simulink model "samples10ANC"  (R2023b)
settings: Solver=FixedStepAuto  StartTime=0.0  StopTime=inf  RelTol=1e-3
model workspace (MAT data in the model file):
  SpF = 10
libraries: matrix_library x22, dspadpt3 x20, raspberrypiAVlib x2, dspfdesign x2
settings Model: ExtModeTrigDuration=2  Creator=aaron  LastModifiedBy=aaron
settings SolverCC: PositivePriorityOrder=on  AutoInsertRateTranBlk=on
settings OptimizationCC: EnhancedBackFolding=on  PassReuseOutputArgsAs=Individual arguments  ZeroExternalMemoryAtStartup=off  ZeroInternalMemoryAtStartup=off  MaxStackSize=64  OptimizeBlockOrder=speed  DifferentSizesBufferReuse=on  OptimizationCustomize=off  EfficientTunableParamExpr=on
settings DebuggingCC: ParameterTunabilityLossMsg=error
settings HardwareCC: ProdBitPerPointer=32  ProdBitPerSizeT=32  ProdBitPerPtrDiffT=32  ProdLargestAtomicInteger=Long  ProdLargestAtomicFloat=Double  ProdWordSize=32  ProdLongLongMode=on  ProdHWDeviceType=ARM Compatible->ARM Cortex
settings RTWCC: Description=Embedded Coder  SystemTargetFile=ert.tlc  HardwareBoard=Raspberry Pi  TLCOptions="-aInlineSetEventsForThisBaseRateFcn=TLC_FALSE -aSuppressMultiTaskScheduler=TLC_FALSE  -aRateBasedStepFcn=0"  TemplateMakefile=ert_default_tmf  Toolchain=GNU GCC Embedded Linux  BuildConfiguration=Faster Runs
settings CodeAppCC: ForceParamTrailComments=on  IgnoreCustomStorageClasses=off  OperatorAnnotations=on  SimulinkDataObjDesc=on  SFDataObjDesc=on  InsertBlockDesc=on
settings ERTTargetCC: SupportVariableSizeSignals=on  ExtModeTransport=2  ExtModeStaticAlloc=on  ExtModeMexFile=ext_xcp  ExtModeIntrfLevel=Level2 - Open

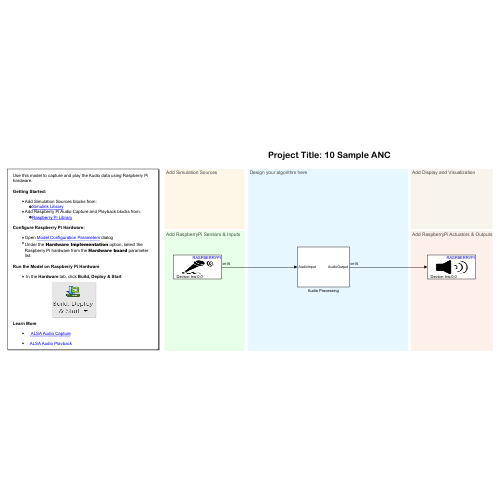
[thumbnail: Simulink's stored preview of the top-level diagram]
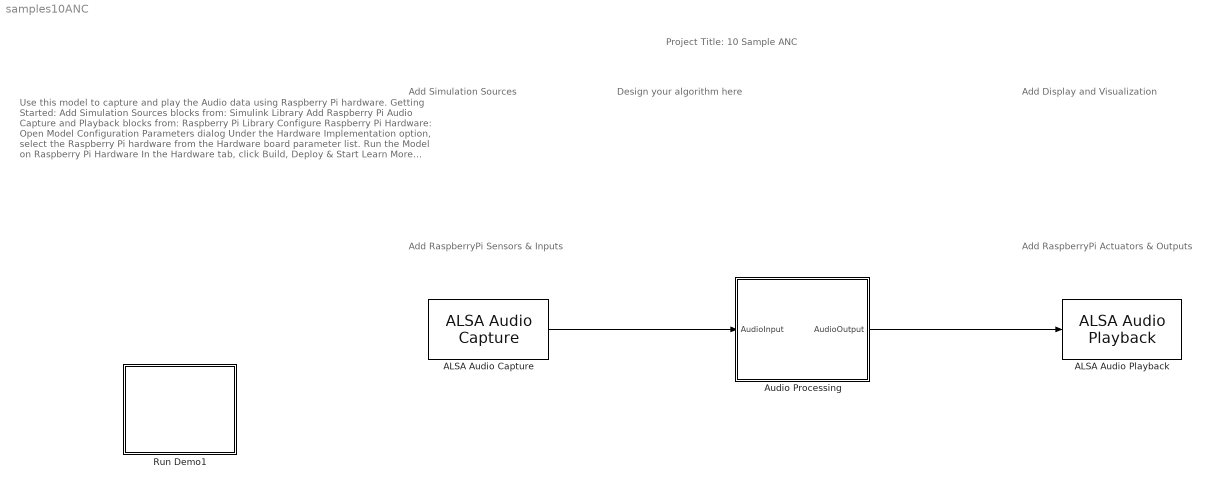
== system samples10ANC ==
  note: Project Title: 10 Sample ANC
  note: Add RaspberryPi Sensors & Inputs
  note: Add Display and Visualization
  note: Add Simulation Sources
  note: Use this model to capture and play the Audio data using Raspberry Pi hardware.
      |
      | Getting Started:
      |
      | Add Simulation Sources blocks from:
      | Simulink Library
      | Add Raspberry Pi Audio Capture and Playback blocks from:
      | Raspberry Pi Library
      |
      | Configure Raspberry Pi Hardware:
      |
      | Open Model Configuration Parameters dialog
      | Under the Hardware Implementation option, select the Raspberry Pi hardware from the Hardware board parameter list.
      |
      | Run the Model on Raspberry Pi Hardware
      |
      | In the Hardware tab, click Build, Deploy & Start
      |
      | Learn More
      | ALSA Audio Capture
      | ALSA Audio Playback
  note: Add RaspberryPi Actuators & Outputs
  note: Design your algorithm here
  ALSA Audio Capture : raspberrypiAVlib/ALSA Audio Capture  deviceStr='hw:0,0'  DataBitDepth=16-bit integer  numberOfChannels=2  sampleRateEnum=44100  frameSize=SpF  QueueDuration=0.5  blockPlatform=Raspberry Pi
  ALSA Audio Playback : raspberrypiAVlib/ALSA Audio Playback  deviceStr='hw:0,0'  sampleRateEnum=44100  queueDuration=0.5  blockPlatform=Raspberry Pi
  Audio Processing : Subsystem
  Run Demo1 : Subsystem  Description=Controls host-side RTDX processing.
      mask Display: pic=imread('raspberrypiBuildDeployAndStart.png');image(pic);
  wires:
  Audio Processing/1(AudioOutput) -> ALSA Audio Playback/1
  ALSA Audio Capture/1 -> Audio Processing/1(AudioInput)

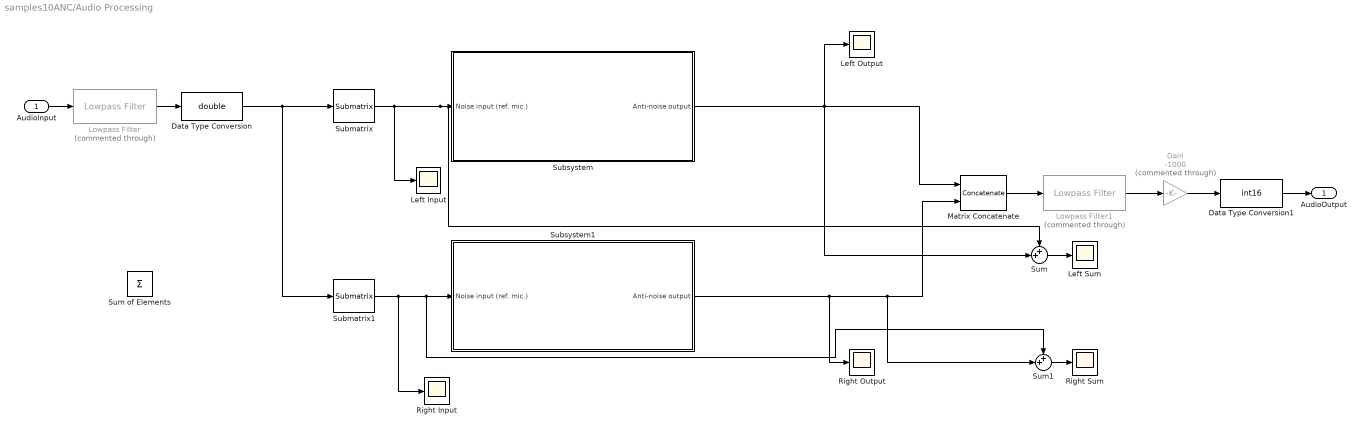
== system samples10ANC/Audio Processing ==
  AudioInput : Inport
  Data Type Conversion : DataTypeConversion  OutDataTypeStr=double  SaturateOnIntegerOverflow=off  RndMeth=Floor
  Data Type Conversion1 : DataTypeConversion  OutDataTypeStr=int16  SaturateOnIntegerOverflow=off  RndMeth=Floor  LockScale=on
  Gain : Gain  Commented=through  Gain=-1000
  Left Input : Scope
  Left Output : Scope
  Left Sum : Scope
  Lowpass Filter : dspfdesign/Lowpass Filter  Commented=through  FilterType=FIR  DesignForMinimumOrder=on  FilterOrder=50  PassbandFrequency=6e2  StopbandFrequency=10e2  PassbandRipple=0.1  StopbandAttenuation=80  SampleRateMode=Specify on dialog  SampleRate=44100  SimulateUsing=Interpreted execution  roundingMode=Floor  coeffsDataTypeStr=fixdt(1,16)
  Lowpass Filter1 : dspfdesign/Lowpass Filter  Commented=through  FilterType=FIR  DesignForMinimumOrder=on  FilterOrder=50  PassbandFrequency=6e2  StopbandFrequency=10e2  PassbandRipple=0.1  StopbandAttenuation=80  SampleRateMode=Specify on dialog  SampleRate=44100  SimulateUsing=Interpreted execution  roundingMode=Floor  coeffsDataTypeStr=fixdt(1,16)
  Matrix Concatenate : Concatenate  Mode=Multidimensional array  ConcatenateDimension=2
  Right Input : Scope
  Right Output : Scope
  Right Sum : Scope
  Submatrix : matrix_library/Submatrix  RowSpan=All rows  RowStartMode=First  RowStartIndex=1  RowEndMode=Last  RowEndIndex=1  ColSpan=One column  ColStartMode=First  ColStartIndex=1  ColEndMode=Last  ColEndIndex=1
  Submatrix1 : matrix_library/Submatrix  RowSpan=All rows  RowStartMode=First  RowStartIndex=1  RowEndMode=Last  RowEndIndex=1  ColSpan=One column  ColStartMode=Last  ColStartIndex=1  ColEndMode=Last  ColEndIndex=1
  Subsystem : Subsystem  TreatAsAtomicUnit=on
  Subsystem1 : Subsystem  TreatAsAtomicUnit=on
  Sum : Sum  Inputs=++|
  Sum of Elements : Sum  Inputs=+
  Sum1 : Sum  Inputs=++|
  AudioOutput : Outport
  wires:
  Data Type Conversion/1 -> Submatrix1/1, Submatrix/1
  Submatrix/1 -> Sum/1, Subsystem/1(Noise input (ref. mic.)), Left Input/1
  AudioInput/1 -> Lowpass Filter/1
  Submatrix1/1 -> Sum1/1, Subsystem1/1(Noise input (ref. mic.)), Right Input/1
  Subsystem1/1(Anti-noise output) -> Sum1/2, Matrix Concatenate/2, Right Output/1
  Lowpass Filter/1 -> Data Type Conversion/1
  Gain/1 -> Data Type Conversion1/1
  Lowpass Filter1/1 -> Gain/1
  Data Type Conversion1/1 -> AudioOutput/1
  Matrix Concatenate/1 -> Lowpass Filter1/1
  Sum1/1 -> Right Sum/1
  Subsystem/1(Anti-noise output) -> Sum/2, Left Output/1, Matrix Concatenate/1
  Sum/1 -> Left Sum/1

== system samples10ANC/Run Demo1 ==

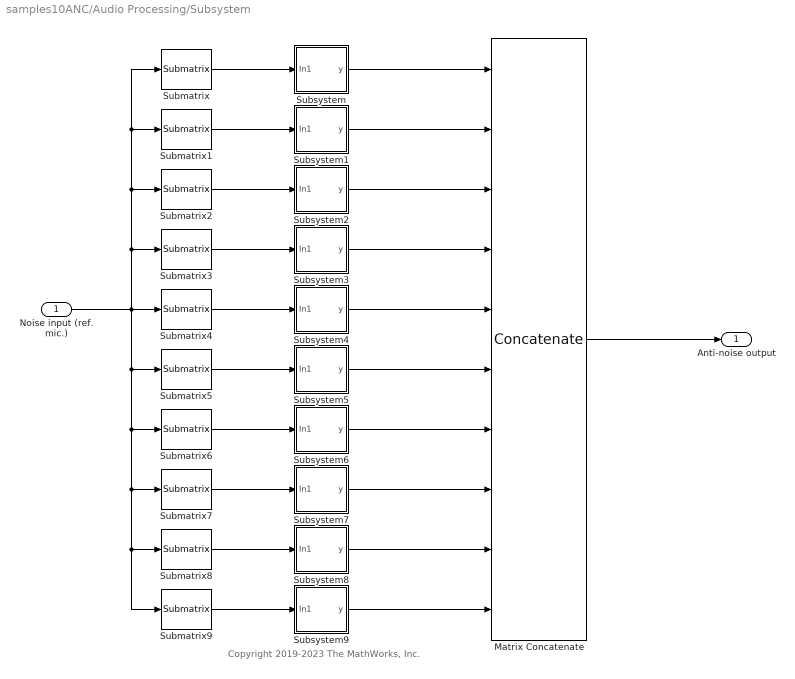
== system samples10ANC/Audio Processing/Subsystem ==
  note: Copyright 2019-2023 The MathWorks, Inc.
  Noise input (ref. mic.) : Inport
  Matrix Concatenate : Concatenate  NumInputs=10  Mode=Multidimensional array
  Submatrix : matrix_library/Submatrix  RowSpan=One row  RowStartMode=Index  RowStartIndex=1  RowEndMode=Last  RowEndIndex=1  ColSpan=One column  ColStartMode=First  ColStartIndex=1  ColEndMode=Last  ColEndIndex=1
  Submatrix1 : matrix_library/Submatrix  RowSpan=One row  RowStartMode=Index  RowStartIndex=2  RowEndMode=Last  RowEndIndex=1  ColSpan=One column  ColStartMode=First  ColStartIndex=1  ColEndMode=Last  ColEndIndex=1
  Submatrix2 : matrix_library/Submatrix  RowSpan=One row  RowStartMode=Index  RowStartIndex=3  RowEndMode=Last  RowEndIndex=1  ColSpan=One column  ColStartMode=First  ColStartIndex=1  ColEndMode=Last  ColEndIndex=1
  Submatrix3 : matrix_library/Submatrix  RowSpan=One row  RowStartMode=Index  RowStartIndex=4  RowEndMode=Last  RowEndIndex=1  ColSpan=One column  ColStartMode=First  ColStartIndex=1  ColEndMode=Last  ColEndIndex=1
  Submatrix4 : matrix_library/Submatrix  RowSpan=One row  RowStartMode=Index  RowStartIndex=5  RowEndMode=Last  RowEndIndex=1  ColSpan=One column  ColStartMode=First  ColStartIndex=1  ColEndMode=Last  ColEndIndex=1
  Submatrix5 : matrix_library/Submatrix  RowSpan=One row  RowStartMode=Index  RowStartIndex=6  RowEndMode=Last  RowEndIndex=1  ColSpan=One column  ColStartMode=First  ColStartIndex=1  ColEndMode=Last  ColEndIndex=1
  Submatrix6 : matrix_library/Submatrix  RowSpan=One row  RowStartMode=Index  RowStartIndex=7  RowEndMode=Last  RowEndIndex=1  ColSpan=One column  ColStartMode=First  ColStartIndex=1  ColEndMode=Last  ColEndIndex=1
  Submatrix7 : matrix_library/Submatrix  RowSpan=One row  RowStartMode=Index  RowStartIndex=8  RowEndMode=Last  RowEndIndex=1  ColSpan=One column  ColStartMode=First  ColStartIndex=1  ColEndMode=Last  ColEndIndex=1
  Submatrix8 : matrix_library/Submatrix  RowSpan=One row  RowStartMode=Index  RowStartIndex=9  RowEndMode=Last  RowEndIndex=1  ColSpan=One column  ColStartMode=First  ColStartIndex=1  ColEndMode=Last  ColEndIndex=1
  Submatrix9 : matrix_library/Submatrix  RowSpan=One row  RowStartMode=Index  RowStartIndex=10  RowEndMode=Last  RowEndIndex=1  ColSpan=One column  ColStartMode=First  ColStartIndex=1  ColEndMode=Last  ColEndIndex=1
  Subsystem : Subsystem
  Subsystem1 : Subsystem
  Subsystem2 : Subsystem
  Subsystem3 : Subsystem
  Subsystem4 : Subsystem
  Subsystem5 : Subsystem
  Subsystem6 : Subsystem
  Subsystem7 : Subsystem
  Subsystem8 : Subsystem
  Subsystem9 : Subsystem
  Anti-noise output : Outport
  wires:
  Submatrix1/1 -> Subsystem1/1(In1)
  Submatrix2/1 -> Subsystem2/1(In1)
  Submatrix3/1 -> Subsystem3/1(In1)
  Submatrix4/1 -> Subsystem4/1(In1)
  Submatrix5/1 -> Subsystem5/1(In1)
  Submatrix6/1 -> Subsystem6/1(In1)
  Submatrix7/1 -> Subsystem7/1(In1)
  Submatrix8/1 -> Subsystem8/1(In1)
  Submatrix9/1 -> Subsystem9/1(In1)
  Noise input (ref. mic.)/1 -> Submatrix9/1, Submatrix8/1, Submatrix7/1, Submatrix6/1, Submatrix5/1, Submatrix/1, Submatrix1/1, Submatrix2/1, Submatrix3/1, Submatrix4/1
  Subsystem1/1(y) -> Matrix Concatenate/2
  Subsystem2/1(y) -> Matrix Concatenate/3
  Subsystem3/1(y) -> Matrix Concatenate/4
  Subsystem4/1(y) -> Matrix Concatenate/5
  Subsystem5/1(y) -> Matrix Concatenate/6
  Matrix Concatenate/1 -> Anti-noise output/1
  Subsystem6/1(y) -> Matrix Concatenate/7
  Subsystem7/1(y) -> Matrix Concatenate/8
  Subsystem8/1(y) -> Matrix Concatenate/9
  Subsystem9/1(y) -> Matrix Concatenate/10
  Submatrix/1 -> Subsystem/1(In1)
  Subsystem/1(y) -> Matrix Concatenate/1

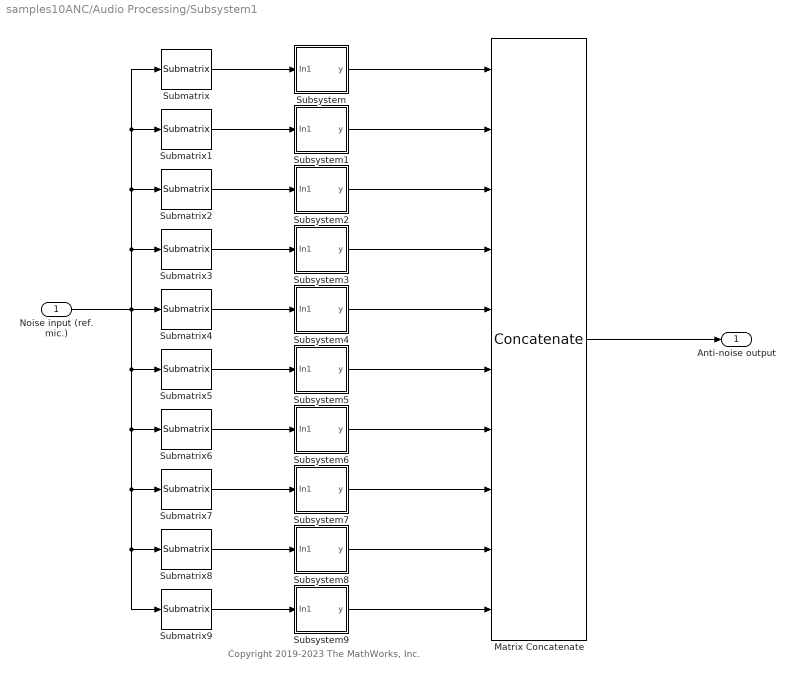
== system samples10ANC/Audio Processing/Subsystem1 ==
  note: Copyright 2019-2023 The MathWorks, Inc.
  Noise input (ref. mic.) : Inport
  Matrix Concatenate : Concatenate  NumInputs=10  Mode=Multidimensional array
  Submatrix : matrix_library/Submatrix  RowSpan=One row  RowStartMode=Index  RowStartIndex=1  RowEndMode=Last  RowEndIndex=1  ColSpan=One column  ColStartMode=First  ColStartIndex=1  ColEndMode=Last  ColEndIndex=1
  Submatrix1 : matrix_library/Submatrix  RowSpan=One row  RowStartMode=Index  RowStartIndex=2  RowEndMode=Last  RowEndIndex=1  ColSpan=One column  ColStartMode=First  ColStartIndex=1  ColEndMode=Last  ColEndIndex=1
  Submatrix2 : matrix_library/Submatrix  RowSpan=One row  RowStartMode=Index  RowStartIndex=3  RowEndMode=Last  RowEndIndex=1  ColSpan=One column  ColStartMode=First  ColStartIndex=1  ColEndMode=Last  ColEndIndex=1
  Submatrix3 : matrix_library/Submatrix  RowSpan=One row  RowStartMode=Index  RowStartIndex=4  RowEndMode=Last  RowEndIndex=1  ColSpan=One column  ColStartMode=First  ColStartIndex=1  ColEndMode=Last  ColEndIndex=1
  Submatrix4 : matrix_library/Submatrix  RowSpan=One row  RowStartMode=Index  RowStartIndex=5  RowEndMode=Last  RowEndIndex=1  ColSpan=One column  ColStartMode=First  ColStartIndex=1  ColEndMode=Last  ColEndIndex=1
  Submatrix5 : matrix_library/Submatrix  RowSpan=One row  RowStartMode=Index  RowStartIndex=6  RowEndMode=Last  RowEndIndex=1  ColSpan=One column  ColStartMode=First  ColStartIndex=1  ColEndMode=Last  ColEndIndex=1
  Submatrix6 : matrix_library/Submatrix  RowSpan=One row  RowStartMode=Index  RowStartIndex=7  RowEndMode=Last  RowEndIndex=1  ColSpan=One column  ColStartMode=First  ColStartIndex=1  ColEndMode=Last  ColEndIndex=1
  Submatrix7 : matrix_library/Submatrix  RowSpan=One row  RowStartMode=Index  RowStartIndex=8  RowEndMode=Last  RowEndIndex=1  ColSpan=One column  ColStartMode=First  ColStartIndex=1  ColEndMode=Last  ColEndIndex=1
  Submatrix8 : matrix_library/Submatrix  RowSpan=One row  RowStartMode=Index  RowStartIndex=9  RowEndMode=Last  RowEndIndex=1  ColSpan=One column  ColStartMode=First  ColStartIndex=1  ColEndMode=Last  ColEndIndex=1
  Submatrix9 : matrix_library/Submatrix  RowSpan=One row  RowStartMode=Index  RowStartIndex=10  RowEndMode=Last  RowEndIndex=1  ColSpan=One column  ColStartMode=First  ColStartIndex=1  ColEndMode=Last  ColEndIndex=1
  Subsystem : Subsystem
  Subsystem1 : Subsystem
  Subsystem2 : Subsystem
  Subsystem3 : Subsystem
  Subsystem4 : Subsystem
  Subsystem5 : Subsystem
  Subsystem6 : Subsystem
  Subsystem7 : Subsystem
  Subsystem8 : Subsystem
  Subsystem9 : Subsystem
  Anti-noise output : Outport
  wires:
  Submatrix1/1 -> Subsystem1/1(In1)
  Submatrix2/1 -> Subsystem2/1(In1)
  Submatrix3/1 -> Subsystem3/1(In1)
  Submatrix4/1 -> Subsystem4/1(In1)
  Submatrix5/1 -> Subsystem5/1(In1)
  Submatrix6/1 -> Subsystem6/1(In1)
  Submatrix7/1 -> Subsystem7/1(In1)
  Submatrix8/1 -> Subsystem8/1(In1)
  Submatrix9/1 -> Subsystem9/1(In1)
  Noise input (ref. mic.)/1 -> Submatrix9/1, Submatrix8/1, Submatrix7/1, Submatrix6/1, Submatrix5/1, Submatrix/1, Submatrix1/1, Submatrix2/1, Submatrix3/1, Submatrix4/1
  Subsystem1/1(y) -> Matrix Concatenate/2
  Subsystem2/1(y) -> Matrix Concatenate/3
  Subsystem3/1(y) -> Matrix Concatenate/4
  Subsystem4/1(y) -> Matrix Concatenate/5
  Subsystem5/1(y) -> Matrix Concatenate/6
  Matrix Concatenate/1 -> Anti-noise output/1
  Subsystem6/1(y) -> Matrix Concatenate/7
  Subsystem7/1(y) -> Matrix Concatenate/8
  Subsystem8/1(y) -> Matrix Concatenate/9
  Subsystem9/1(y) -> Matrix Concatenate/10
  Submatrix/1 -> Subsystem/1(In1)
  Subsystem/1(y) -> Matrix Concatenate/1

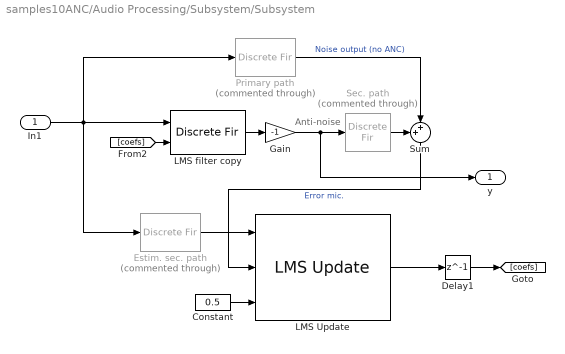
== system samples10ANC/Audio Processing/Subsystem/Subsystem ==
  note: Anti-noise
  In1 : Inport
  Constant : Constant  Value=0.5
  Delay1 : Delay  DelayLength=1
  Estim. sec. path : DiscreteFir  Commented=through  Coefficients="[0.466  0.533  -0.257  -0.274  -0.231  -0.175]"
  Gain : Gain  Gain=-1
  LMS Update : dspadpt3/LMS Update  Method=Normalized LMS  Length=200  NumFilters=1  StepSizeSource=Input port  StepSize=0.1  LeakageFactor=1.0  InitialConditions=0  AdaptiveFilterMode=Tapped delay-line FIR filter  EnableAdaptInput=off  EnableResetInput=off  SimulateUsing=Interpreted execution
  LMS filter copy : DiscreteFir  CoefSource=Input port
      settings: InputPortMap=u0,u1
  Primary path : DiscreteFir  Commented=through  Coefficients=conv([0.5 0.5 -.3 -.3 -.2 -.2],[.1 -.1 .2 -.2 .3 -.3 .15 -.15])
  Sec. path : DiscreteFir  Commented=through  Coefficients=[0.5 0.5 -.3 -.3 -.2 -.2]
  Sum : Sum  Inputs=++|
  y : Outport
  wires:
  Primary path/1 -> Sum/2  "Noise output (no ANC)"
  Gain/1 -> y/1, Sec. path/1
  Constant/1 -> LMS Update/3
  LMS filter copy/1 -> Gain/1
  [coefs] -> LMS filter copy/2
  Sum/1 -> LMS Update/2  "Error mic."
  Delay1/1 -> [coefs]
  LMS Update/1 -> Delay1/1
  In1/1 -> Primary path/1, Estim. sec. path/1, LMS filter copy/1
  Estim. sec. path/1 -> LMS Update/1
  Sec. path/1 -> Sum/1

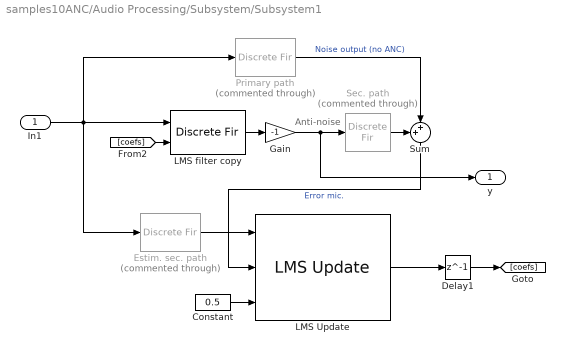
== system samples10ANC/Audio Processing/Subsystem/Subsystem1 ==
  note: Anti-noise
  In1 : Inport
  Constant : Constant  Value=0.5
  Delay1 : Delay  DelayLength=1
  Estim. sec. path : DiscreteFir  Commented=through  Coefficients="[0.466  0.533  -0.257  -0.274  -0.231  -0.175]"
  Gain : Gain  Gain=-1
  LMS Update : dspadpt3/LMS Update  Method=Normalized LMS  Length=200  NumFilters=1  StepSizeSource=Input port  StepSize=0.1  LeakageFactor=1.0  InitialConditions=0  AdaptiveFilterMode=Tapped delay-line FIR filter  EnableAdaptInput=off  EnableResetInput=off  SimulateUsing=Interpreted execution
  LMS filter copy : DiscreteFir  CoefSource=Input port
      settings: InputPortMap=u0,u1
  Primary path : DiscreteFir  Commented=through  Coefficients=conv([0.5 0.5 -.3 -.3 -.2 -.2],[.1 -.1 .2 -.2 .3 -.3 .15 -.15])
  Sec. path : DiscreteFir  Commented=through  Coefficients=[0.5 0.5 -.3 -.3 -.2 -.2]
  Sum : Sum  Inputs=++|
  y : Outport
  wires:
  Primary path/1 -> Sum/2  "Noise output (no ANC)"
  Gain/1 -> y/1, Sec. path/1
  Constant/1 -> LMS Update/3
  LMS filter copy/1 -> Gain/1
  [coefs] -> LMS filter copy/2
  Sum/1 -> LMS Update/2  "Error mic."
  Delay1/1 -> [coefs]
  LMS Update/1 -> Delay1/1
  In1/1 -> Primary path/1, Estim. sec. path/1, LMS filter copy/1
  Estim. sec. path/1 -> LMS Update/1
  Sec. path/1 -> Sum/1

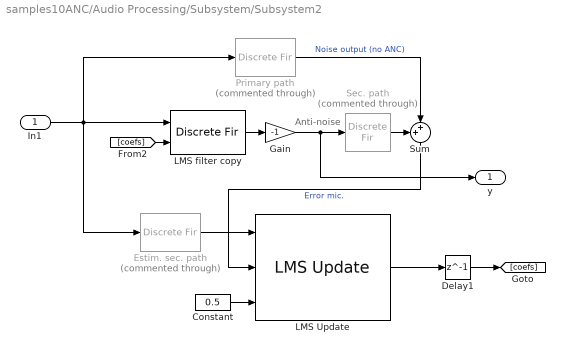
== system samples10ANC/Audio Processing/Subsystem/Subsystem2 ==
  note: Anti-noise
  In1 : Inport
  Constant : Constant  Value=0.5
  Delay1 : Delay  DelayLength=1
  Estim. sec. path : DiscreteFir  Commented=through  Coefficients="[0.466  0.533  -0.257  -0.274  -0.231  -0.175]"
  Gain : Gain  Gain=-1
  LMS Update : dspadpt3/LMS Update  Method=Normalized LMS  Length=200  NumFilters=1  StepSizeSource=Input port  StepSize=0.1  LeakageFactor=1.0  InitialConditions=0  AdaptiveFilterMode=Tapped delay-line FIR filter  EnableAdaptInput=off  EnableResetInput=off  SimulateUsing=Interpreted execution
  LMS filter copy : DiscreteFir  CoefSource=Input port
      settings: InputPortMap=u0,u1
  Primary path : DiscreteFir  Commented=through  Coefficients=conv([0.5 0.5 -.3 -.3 -.2 -.2],[.1 -.1 .2 -.2 .3 -.3 .15 -.15])
  Sec. path : DiscreteFir  Commented=through  Coefficients=[0.5 0.5 -.3 -.3 -.2 -.2]
  Sum : Sum  Inputs=++|
  y : Outport
  wires:
  Primary path/1 -> Sum/2  "Noise output (no ANC)"
  Gain/1 -> y/1, Sec. path/1
  Constant/1 -> LMS Update/3
  LMS filter copy/1 -> Gain/1
  [coefs] -> LMS filter copy/2
  Sum/1 -> LMS Update/2  "Error mic."
  Delay1/1 -> [coefs]
  LMS Update/1 -> Delay1/1
  In1/1 -> Primary path/1, Estim. sec. path/1, LMS filter copy/1
  Estim. sec. path/1 -> LMS Update/1
  Sec. path/1 -> Sum/1

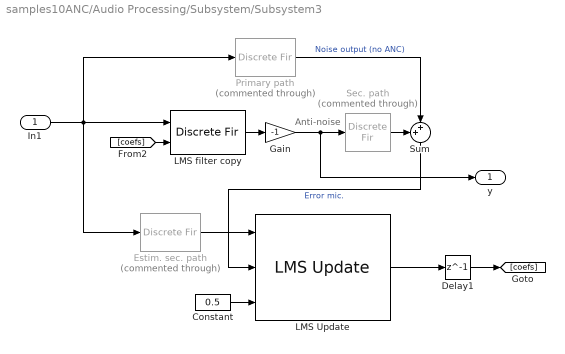
== system samples10ANC/Audio Processing/Subsystem/Subsystem3 ==
  note: Anti-noise
  In1 : Inport
  Constant : Constant  Value=0.5
  Delay1 : Delay  DelayLength=1
  Estim. sec. path : DiscreteFir  Commented=through  Coefficients="[0.466  0.533  -0.257  -0.274  -0.231  -0.175]"
  Gain : Gain  Gain=-1
  LMS Update : dspadpt3/LMS Update  Method=Normalized LMS  Length=200  NumFilters=1  StepSizeSource=Input port  StepSize=0.1  LeakageFactor=1.0  InitialConditions=0  AdaptiveFilterMode=Tapped delay-line FIR filter  EnableAdaptInput=off  EnableResetInput=off  SimulateUsing=Interpreted execution
  LMS filter copy : DiscreteFir  CoefSource=Input port
      settings: InputPortMap=u0,u1
  Primary path : DiscreteFir  Commented=through  Coefficients=conv([0.5 0.5 -.3 -.3 -.2 -.2],[.1 -.1 .2 -.2 .3 -.3 .15 -.15])
  Sec. path : DiscreteFir  Commented=through  Coefficients=[0.5 0.5 -.3 -.3 -.2 -.2]
  Sum : Sum  Inputs=++|
  y : Outport
  wires:
  Primary path/1 -> Sum/2  "Noise output (no ANC)"
  Gain/1 -> y/1, Sec. path/1
  Constant/1 -> LMS Update/3
  LMS filter copy/1 -> Gain/1
  [coefs] -> LMS filter copy/2
  Sum/1 -> LMS Update/2  "Error mic."
  Delay1/1 -> [coefs]
  LMS Update/1 -> Delay1/1
  In1/1 -> Primary path/1, Estim. sec. path/1, LMS filter copy/1
  Estim. sec. path/1 -> LMS Update/1
  Sec. path/1 -> Sum/1

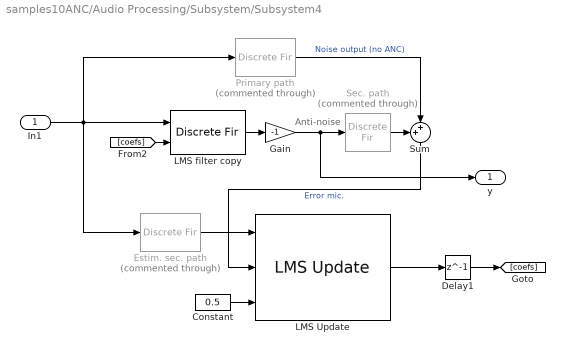
== system samples10ANC/Audio Processing/Subsystem/Subsystem4 ==
  note: Anti-noise
  In1 : Inport
  Constant : Constant  Value=0.5
  Delay1 : Delay  DelayLength=1
  Estim. sec. path : DiscreteFir  Commented=through  Coefficients="[0.466  0.533  -0.257  -0.274  -0.231  -0.175]"
  Gain : Gain  Gain=-1
  LMS Update : dspadpt3/LMS Update  Method=Normalized LMS  Length=200  NumFilters=1  StepSizeSource=Input port  StepSize=0.1  LeakageFactor=1.0  InitialConditions=0  AdaptiveFilterMode=Tapped delay-line FIR filter  EnableAdaptInput=off  EnableResetInput=off  SimulateUsing=Interpreted execution
  LMS filter copy : DiscreteFir  CoefSource=Input port
      settings: InputPortMap=u0,u1
  Primary path : DiscreteFir  Commented=through  Coefficients=conv([0.5 0.5 -.3 -.3 -.2 -.2],[.1 -.1 .2 -.2 .3 -.3 .15 -.15])
  Sec. path : DiscreteFir  Commented=through  Coefficients=[0.5 0.5 -.3 -.3 -.2 -.2]
  Sum : Sum  Inputs=++|
  y : Outport
  wires:
  Primary path/1 -> Sum/2  "Noise output (no ANC)"
  Gain/1 -> y/1, Sec. path/1
  Constant/1 -> LMS Update/3
  LMS filter copy/1 -> Gain/1
  [coefs] -> LMS filter copy/2
  Sum/1 -> LMS Update/2  "Error mic."
  Delay1/1 -> [coefs]
  LMS Update/1 -> Delay1/1
  In1/1 -> Primary path/1, Estim. sec. path/1, LMS filter copy/1
  Estim. sec. path/1 -> LMS Update/1
  Sec. path/1 -> Sum/1

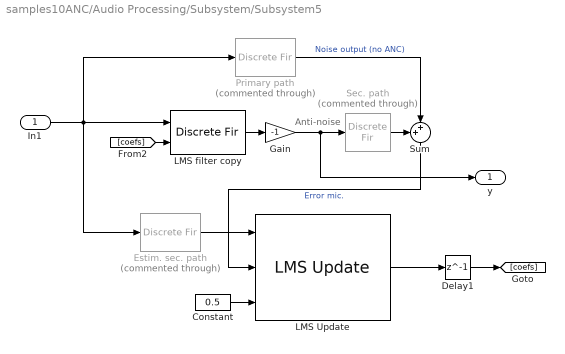
== system samples10ANC/Audio Processing/Subsystem/Subsystem5 ==
  note: Anti-noise
  In1 : Inport
  Constant : Constant  Value=0.5
  Delay1 : Delay  DelayLength=1
  Estim. sec. path : DiscreteFir  Commented=through  Coefficients="[0.466  0.533  -0.257  -0.274  -0.231  -0.175]"
  Gain : Gain  Gain=-1
  LMS Update : dspadpt3/LMS Update  Method=Normalized LMS  Length=200  NumFilters=1  StepSizeSource=Input port  StepSize=0.1  LeakageFactor=1.0  InitialConditions=0  AdaptiveFilterMode=Tapped delay-line FIR filter  EnableAdaptInput=off  EnableResetInput=off  SimulateUsing=Interpreted execution
  LMS filter copy : DiscreteFir  CoefSource=Input port
      settings: InputPortMap=u0,u1
  Primary path : DiscreteFir  Commented=through  Coefficients=conv([0.5 0.5 -.3 -.3 -.2 -.2],[.1 -.1 .2 -.2 .3 -.3 .15 -.15])
  Sec. path : DiscreteFir  Commented=through  Coefficients=[0.5 0.5 -.3 -.3 -.2 -.2]
  Sum : Sum  Inputs=++|
  y : Outport
  wires:
  Primary path/1 -> Sum/2  "Noise output (no ANC)"
  Gain/1 -> y/1, Sec. path/1
  Constant/1 -> LMS Update/3
  LMS filter copy/1 -> Gain/1
  [coefs] -> LMS filter copy/2
  Sum/1 -> LMS Update/2  "Error mic."
  Delay1/1 -> [coefs]
  LMS Update/1 -> Delay1/1
  In1/1 -> Primary path/1, Estim. sec. path/1, LMS filter copy/1
  Estim. sec. path/1 -> LMS Update/1
  Sec. path/1 -> Sum/1

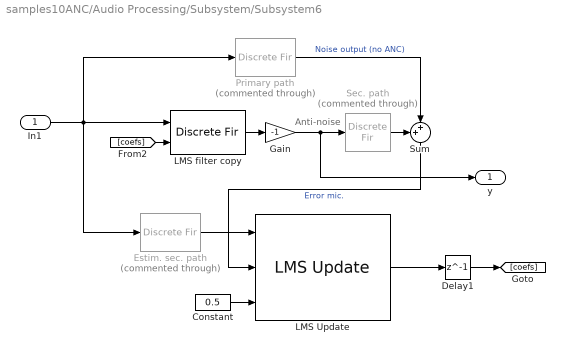
== system samples10ANC/Audio Processing/Subsystem/Subsystem6 ==
  note: Anti-noise
  In1 : Inport
  Constant : Constant  Value=0.5
  Delay1 : Delay  DelayLength=1
  Estim. sec. path : DiscreteFir  Commented=through  Coefficients="[0.466  0.533  -0.257  -0.274  -0.231  -0.175]"
  Gain : Gain  Gain=-1
  LMS Update : dspadpt3/LMS Update  Method=Normalized LMS  Length=200  NumFilters=1  StepSizeSource=Input port  StepSize=0.1  LeakageFactor=1.0  InitialConditions=0  AdaptiveFilterMode=Tapped delay-line FIR filter  EnableAdaptInput=off  EnableResetInput=off  SimulateUsing=Interpreted execution
  LMS filter copy : DiscreteFir  CoefSource=Input port
      settings: InputPortMap=u0,u1
  Primary path : DiscreteFir  Commented=through  Coefficients=conv([0.5 0.5 -.3 -.3 -.2 -.2],[.1 -.1 .2 -.2 .3 -.3 .15 -.15])
  Sec. path : DiscreteFir  Commented=through  Coefficients=[0.5 0.5 -.3 -.3 -.2 -.2]
  Sum : Sum  Inputs=++|
  y : Outport
  wires:
  Primary path/1 -> Sum/2  "Noise output (no ANC)"
  Gain/1 -> y/1, Sec. path/1
  Constant/1 -> LMS Update/3
  LMS filter copy/1 -> Gain/1
  [coefs] -> LMS filter copy/2
  Sum/1 -> LMS Update/2  "Error mic."
  Delay1/1 -> [coefs]
  LMS Update/1 -> Delay1/1
  In1/1 -> Primary path/1, Estim. sec. path/1, LMS filter copy/1
  Estim. sec. path/1 -> LMS Update/1
  Sec. path/1 -> Sum/1

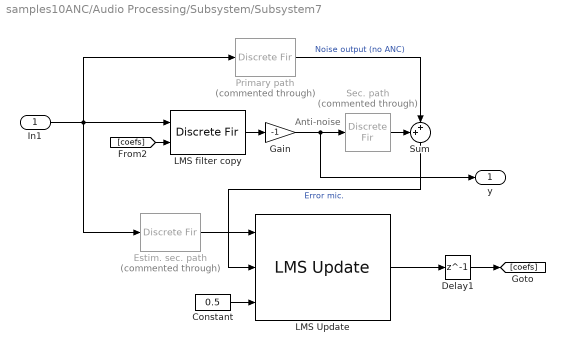
== system samples10ANC/Audio Processing/Subsystem/Subsystem7 ==
  note: Anti-noise
  In1 : Inport
  Constant : Constant  Value=0.5
  Delay1 : Delay  DelayLength=1
  Estim. sec. path : DiscreteFir  Commented=through  Coefficients="[0.466  0.533  -0.257  -0.274  -0.231  -0.175]"
  Gain : Gain  Gain=-1
  LMS Update : dspadpt3/LMS Update  Method=Normalized LMS  Length=200  NumFilters=1  StepSizeSource=Input port  StepSize=0.1  LeakageFactor=1.0  InitialConditions=0  AdaptiveFilterMode=Tapped delay-line FIR filter  EnableAdaptInput=off  EnableResetInput=off  SimulateUsing=Interpreted execution
  LMS filter copy : DiscreteFir  CoefSource=Input port
      settings: InputPortMap=u0,u1
  Primary path : DiscreteFir  Commented=through  Coefficients=conv([0.5 0.5 -.3 -.3 -.2 -.2],[.1 -.1 .2 -.2 .3 -.3 .15 -.15])
  Sec. path : DiscreteFir  Commented=through  Coefficients=[0.5 0.5 -.3 -.3 -.2 -.2]
  Sum : Sum  Inputs=++|
  y : Outport
  wires:
  Primary path/1 -> Sum/2  "Noise output (no ANC)"
  Gain/1 -> y/1, Sec. path/1
  Constant/1 -> LMS Update/3
  LMS filter copy/1 -> Gain/1
  [coefs] -> LMS filter copy/2
  Sum/1 -> LMS Update/2  "Error mic."
  Delay1/1 -> [coefs]
  LMS Update/1 -> Delay1/1
  In1/1 -> Primary path/1, Estim. sec. path/1, LMS filter copy/1
  Estim. sec. path/1 -> LMS Update/1
  Sec. path/1 -> Sum/1

== system samples10ANC/Audio Processing/Subsystem/Subsystem8 ==
  note: Anti-noise
  In1 : Inport
  Constant : Constant  Value=0.5
  Delay1 : Delay  DelayLength=1
  Estim. sec. path : DiscreteFir  Commented=through  Coefficients="[0.466  0.533  -0.257  -0.274  -0.231  -0.175]"
  Gain : Gain  Gain=-1
  LMS Update : dspadpt3/LMS Update  Method=Normalized LMS  Length=200  NumFilters=1  StepSizeSource=Input port  StepSize=0.1  LeakageFactor=1.0  InitialConditions=0  AdaptiveFilterMode=Tapped delay-line FIR filter  EnableAdaptInput=off  EnableResetInput=off  SimulateUsing=Interpreted execution
  LMS filter copy : DiscreteFir  CoefSource=Input port
      settings: InputPortMap=u0,u1
  Primary path : DiscreteFir  Commented=through  Coefficients=conv([0.5 0.5 -.3 -.3 -.2 -.2],[.1 -.1 .2 -.2 .3 -.3 .15 -.15])
  Sec. path : DiscreteFir  Commented=through  Coefficients=[0.5 0.5 -.3 -.3 -.2 -.2]
  Sum : Sum  Inputs=++|
  y : Outport
  wires:
  Primary path/1 -> Sum/2  "Noise output (no ANC)"
  Gain/1 -> y/1, Sec. path/1
  Constant/1 -> LMS Update/3
  LMS filter copy/1 -> Gain/1
  [coefs] -> LMS filter copy/2
  Sum/1 -> LMS Update/2  "Error mic."
  Delay1/1 -> [coefs]
  LMS Update/1 -> Delay1/1
  In1/1 -> Primary path/1, Estim. sec. path/1, LMS filter copy/1
  Estim. sec. path/1 -> LMS Update/1
  Sec. path/1 -> Sum/1

== system samples10ANC/Audio Processing/Subsystem/Subsystem9 ==
  note: Anti-noise
  In1 : Inport
  Constant : Constant  Value=0.5
  Delay1 : Delay  DelayLength=1
  Estim. sec. path : DiscreteFir  Commented=through  Coefficients="[0.466  0.533  -0.257  -0.274  -0.231  -0.175]"
  Gain : Gain  Gain=-1
  LMS Update : dspadpt3/LMS Update  Method=Normalized LMS  Length=200  NumFilters=1  StepSizeSource=Input port  StepSize=0.1  LeakageFactor=1.0  InitialConditions=0  AdaptiveFilterMode=Tapped delay-line FIR filter  EnableAdaptInput=off  EnableResetInput=off  SimulateUsing=Interpreted execution
  LMS filter copy : DiscreteFir  CoefSource=Input port
      settings: InputPortMap=u0,u1
  Primary path : DiscreteFir  Commented=through  Coefficients=conv([0.5 0.5 -.3 -.3 -.2 -.2],[.1 -.1 .2 -.2 .3 -.3 .15 -.15])
  Sec. path : DiscreteFir  Commented=through  Coefficients=[0.5 0.5 -.3 -.3 -.2 -.2]
  Sum : Sum  Inputs=++|
  y : Outport
  wires:
  Primary path/1 -> Sum/2  "Noise output (no ANC)"
  Gain/1 -> y/1, Sec. path/1
  Constant/1 -> LMS Update/3
  LMS filter copy/1 -> Gain/1
  [coefs] -> LMS filter copy/2
  Sum/1 -> LMS Update/2  "Error mic."
  Delay1/1 -> [coefs]
  LMS Update/1 -> Delay1/1
  In1/1 -> Primary path/1, Estim. sec. path/1, LMS filter copy/1
  Estim. sec. path/1 -> LMS Update/1
  Sec. path/1 -> Sum/1

== system samples10ANC/Audio Processing/Subsystem1/Subsystem ==
  note: Anti-noise
  In1 : Inport
  Constant : Constant  Value=0.5
  Delay1 : Delay  DelayLength=1
  Estim. sec. path : DiscreteFir  Commented=through  Coefficients="[0.466  0.533  -0.257  -0.274  -0.231  -0.175]"
  Gain : Gain  Gain=-1
  LMS Update : dspadpt3/LMS Update  Method=Normalized LMS  Length=200  NumFilters=1  StepSizeSource=Input port  StepSize=0.1  LeakageFactor=1.0  InitialConditions=0  AdaptiveFilterMode=Tapped delay-line FIR filter  EnableAdaptInput=off  EnableResetInput=off  SimulateUsing=Interpreted execution
  LMS filter copy : DiscreteFir  CoefSource=Input port
      settings: InputPortMap=u0,u1
  Primary path : DiscreteFir  Commented=through  Coefficients=conv([0.5 0.5 -.3 -.3 -.2 -.2],[.1 -.1 .2 -.2 .3 -.3 .15 -.15])
  Sec. path : DiscreteFir  Commented=through  Coefficients=[0.5 0.5 -.3 -.3 -.2 -.2]
  Sum : Sum  Inputs=++|
  y : Outport
  wires:
  Primary path/1 -> Sum/2  "Noise output (no ANC)"
  Gain/1 -> y/1, Sec. path/1
  Constant/1 -> LMS Update/3
  LMS filter copy/1 -> Gain/1
  [coefs] -> LMS filter copy/2
  Sum/1 -> LMS Update/2  "Error mic."
  Delay1/1 -> [coefs]
  LMS Update/1 -> Delay1/1
  In1/1 -> Primary path/1, Estim. sec. path/1, LMS filter copy/1
  Estim. sec. path/1 -> LMS Update/1
  Sec. path/1 -> Sum/1

== system samples10ANC/Audio Processing/Subsystem1/Subsystem1 ==
  note: Anti-noise
  In1 : Inport
  Constant : Constant  Value=0.5
  Delay1 : Delay  DelayLength=1
  Estim. sec. path : DiscreteFir  Commented=through  Coefficients="[0.466  0.533  -0.257  -0.274  -0.231  -0.175]"
  Gain : Gain  Gain=-1
  LMS Update : dspadpt3/LMS Update  Method=Normalized LMS  Length=200  NumFilters=1  StepSizeSource=Input port  StepSize=0.1  LeakageFactor=1.0  InitialConditions=0  AdaptiveFilterMode=Tapped delay-line FIR filter  EnableAdaptInput=off  EnableResetInput=off  SimulateUsing=Interpreted execution
  LMS filter copy : DiscreteFir  CoefSource=Input port
      settings: InputPortMap=u0,u1
  Primary path : DiscreteFir  Commented=through  Coefficients=conv([0.5 0.5 -.3 -.3 -.2 -.2],[.1 -.1 .2 -.2 .3 -.3 .15 -.15])
  Sec. path : DiscreteFir  Commented=through  Coefficients=[0.5 0.5 -.3 -.3 -.2 -.2]
  Sum : Sum  Inputs=++|
  y : Outport
  wires:
  Primary path/1 -> Sum/2  "Noise output (no ANC)"
  Gain/1 -> y/1, Sec. path/1
  Constant/1 -> LMS Update/3
  LMS filter copy/1 -> Gain/1
  [coefs] -> LMS filter copy/2
  Sum/1 -> LMS Update/2  "Error mic."
  Delay1/1 -> [coefs]
  LMS Update/1 -> Delay1/1
  In1/1 -> Primary path/1, Estim. sec. path/1, LMS filter copy/1
  Estim. sec. path/1 -> LMS Update/1
  Sec. path/1 -> Sum/1

== system samples10ANC/Audio Processing/Subsystem1/Subsystem2 ==
  note: Anti-noise
  In1 : Inport
  Constant : Constant  Value=0.5
  Delay1 : Delay  DelayLength=1
  Estim. sec. path : DiscreteFir  Commented=through  Coefficients="[0.466  0.533  -0.257  -0.274  -0.231  -0.175]"
  Gain : Gain  Gain=-1
  LMS Update : dspadpt3/LMS Update  Method=Normalized LMS  Length=200  NumFilters=1  StepSizeSource=Input port  StepSize=0.1  LeakageFactor=1.0  InitialConditions=0  AdaptiveFilterMode=Tapped delay-line FIR filter  EnableAdaptInput=off  EnableResetInput=off  SimulateUsing=Interpreted execution
  LMS filter copy : DiscreteFir  CoefSource=Input port
      settings: InputPortMap=u0,u1
  Primary path : DiscreteFir  Commented=through  Coefficients=conv([0.5 0.5 -.3 -.3 -.2 -.2],[.1 -.1 .2 -.2 .3 -.3 .15 -.15])
  Sec. path : DiscreteFir  Commented=through  Coefficients=[0.5 0.5 -.3 -.3 -.2 -.2]
  Sum : Sum  Inputs=++|
  y : Outport
  wires:
  Primary path/1 -> Sum/2  "Noise output (no ANC)"
  Gain/1 -> y/1, Sec. path/1
  Constant/1 -> LMS Update/3
  LMS filter copy/1 -> Gain/1
  [coefs] -> LMS filter copy/2
  Sum/1 -> LMS Update/2  "Error mic."
  Delay1/1 -> [coefs]
  LMS Update/1 -> Delay1/1
  In1/1 -> Primary path/1, Estim. sec. path/1, LMS filter copy/1
  Estim. sec. path/1 -> LMS Update/1
  Sec. path/1 -> Sum/1

== system samples10ANC/Audio Processing/Subsystem1/Subsystem3 ==
  note: Anti-noise
  In1 : Inport
  Constant : Constant  Value=0.5
  Delay1 : Delay  DelayLength=1
  Estim. sec. path : DiscreteFir  Commented=through  Coefficients="[0.466  0.533  -0.257  -0.274  -0.231  -0.175]"
  Gain : Gain  Gain=-1
  LMS Update : dspadpt3/LMS Update  Method=Normalized LMS  Length=200  NumFilters=1  StepSizeSource=Input port  StepSize=0.1  LeakageFactor=1.0  InitialConditions=0  AdaptiveFilterMode=Tapped delay-line FIR filter  EnableAdaptInput=off  EnableResetInput=off  SimulateUsing=Interpreted execution
  LMS filter copy : DiscreteFir  CoefSource=Input port
      settings: InputPortMap=u0,u1
  Primary path : DiscreteFir  Commented=through  Coefficients=conv([0.5 0.5 -.3 -.3 -.2 -.2],[.1 -.1 .2 -.2 .3 -.3 .15 -.15])
  Sec. path : DiscreteFir  Commented=through  Coefficients=[0.5 0.5 -.3 -.3 -.2 -.2]
  Sum : Sum  Inputs=++|
  y : Outport
  wires:
  Primary path/1 -> Sum/2  "Noise output (no ANC)"
  Gain/1 -> y/1, Sec. path/1
  Constant/1 -> LMS Update/3
  LMS filter copy/1 -> Gain/1
  [coefs] -> LMS filter copy/2
  Sum/1 -> LMS Update/2  "Error mic."
  Delay1/1 -> [coefs]
  LMS Update/1 -> Delay1/1
  In1/1 -> Primary path/1, Estim. sec. path/1, LMS filter copy/1
  Estim. sec. path/1 -> LMS Update/1
  Sec. path/1 -> Sum/1

== system samples10ANC/Audio Processing/Subsystem1/Subsystem4 ==
  note: Anti-noise
  In1 : Inport
  Constant : Constant  Value=0.5
  Delay1 : Delay  DelayLength=1
  Estim. sec. path : DiscreteFir  Commented=through  Coefficients="[0.466  0.533  -0.257  -0.274  -0.231  -0.175]"
  Gain : Gain  Gain=-1
  LMS Update : dspadpt3/LMS Update  Method=Normalized LMS  Length=200  NumFilters=1  StepSizeSource=Input port  StepSize=0.1  LeakageFactor=1.0  InitialConditions=0  AdaptiveFilterMode=Tapped delay-line FIR filter  EnableAdaptInput=off  EnableResetInput=off  SimulateUsing=Interpreted execution
  LMS filter copy : DiscreteFir  CoefSource=Input port
      settings: InputPortMap=u0,u1
  Primary path : DiscreteFir  Commented=through  Coefficients=conv([0.5 0.5 -.3 -.3 -.2 -.2],[.1 -.1 .2 -.2 .3 -.3 .15 -.15])
  Sec. path : DiscreteFir  Commented=through  Coefficients=[0.5 0.5 -.3 -.3 -.2 -.2]
  Sum : Sum  Inputs=++|
  y : Outport
  wires:
  Primary path/1 -> Sum/2  "Noise output (no ANC)"
  Gain/1 -> y/1, Sec. path/1
  Constant/1 -> LMS Update/3
  LMS filter copy/1 -> Gain/1
  [coefs] -> LMS filter copy/2
  Sum/1 -> LMS Update/2  "Error mic."
  Delay1/1 -> [coefs]
  LMS Update/1 -> Delay1/1
  In1/1 -> Primary path/1, Estim. sec. path/1, LMS filter copy/1
  Estim. sec. path/1 -> LMS Update/1
  Sec. path/1 -> Sum/1

== system samples10ANC/Audio Processing/Subsystem1/Subsystem5 ==
  note: Anti-noise
  In1 : Inport
  Constant : Constant  Value=0.5
  Delay1 : Delay  DelayLength=1
  Estim. sec. path : DiscreteFir  Commented=through  Coefficients="[0.466  0.533  -0.257  -0.274  -0.231  -0.175]"
  Gain : Gain  Gain=-1
  LMS Update : dspadpt3/LMS Update  Method=Normalized LMS  Length=200  NumFilters=1  StepSizeSource=Input port  StepSize=0.1  LeakageFactor=1.0  InitialConditions=0  AdaptiveFilterMode=Tapped delay-line FIR filter  EnableAdaptInput=off  EnableResetInput=off  SimulateUsing=Interpreted execution
  LMS filter copy : DiscreteFir  CoefSource=Input port
      settings: InputPortMap=u0,u1
  Primary path : DiscreteFir  Commented=through  Coefficients=conv([0.5 0.5 -.3 -.3 -.2 -.2],[.1 -.1 .2 -.2 .3 -.3 .15 -.15])
  Sec. path : DiscreteFir  Commented=through  Coefficients=[0.5 0.5 -.3 -.3 -.2 -.2]
  Sum : Sum  Inputs=++|
  y : Outport
  wires:
  Primary path/1 -> Sum/2  "Noise output (no ANC)"
  Gain/1 -> y/1, Sec. path/1
  Constant/1 -> LMS Update/3
  LMS filter copy/1 -> Gain/1
  [coefs] -> LMS filter copy/2
  Sum/1 -> LMS Update/2  "Error mic."
  Delay1/1 -> [coefs]
  LMS Update/1 -> Delay1/1
  In1/1 -> Primary path/1, Estim. sec. path/1, LMS filter copy/1
  Estim. sec. path/1 -> LMS Update/1
  Sec. path/1 -> Sum/1

== system samples10ANC/Audio Processing/Subsystem1/Subsystem6 ==
  note: Anti-noise
  In1 : Inport
  Constant : Constant  Value=0.5
  Delay1 : Delay  DelayLength=1
  Estim. sec. path : DiscreteFir  Commented=through  Coefficients="[0.466  0.533  -0.257  -0.274  -0.231  -0.175]"
  Gain : Gain  Gain=-1
  LMS Update : dspadpt3/LMS Update  Method=Normalized LMS  Length=200  NumFilters=1  StepSizeSource=Input port  StepSize=0.1  LeakageFactor=1.0  InitialConditions=0  AdaptiveFilterMode=Tapped delay-line FIR filter  EnableAdaptInput=off  EnableResetInput=off  SimulateUsing=Interpreted execution
  LMS filter copy : DiscreteFir  CoefSource=Input port
      settings: InputPortMap=u0,u1
  Primary path : DiscreteFir  Commented=through  Coefficients=conv([0.5 0.5 -.3 -.3 -.2 -.2],[.1 -.1 .2 -.2 .3 -.3 .15 -.15])
  Sec. path : DiscreteFir  Commented=through  Coefficients=[0.5 0.5 -.3 -.3 -.2 -.2]
  Sum : Sum  Inputs=++|
  y : Outport
  wires:
  Primary path/1 -> Sum/2  "Noise output (no ANC)"
  Gain/1 -> y/1, Sec. path/1
  Constant/1 -> LMS Update/3
  LMS filter copy/1 -> Gain/1
  [coefs] -> LMS filter copy/2
  Sum/1 -> LMS Update/2  "Error mic."
  Delay1/1 -> [coefs]
  LMS Update/1 -> Delay1/1
  In1/1 -> Primary path/1, Estim. sec. path/1, LMS filter copy/1
  Estim. sec. path/1 -> LMS Update/1
  Sec. path/1 -> Sum/1

== system samples10ANC/Audio Processing/Subsystem1/Subsystem7 ==
  note: Anti-noise
  In1 : Inport
  Constant : Constant  Value=0.5
  Delay1 : Delay  DelayLength=1
  Estim. sec. path : DiscreteFir  Commented=through  Coefficients="[0.466  0.533  -0.257  -0.274  -0.231  -0.175]"
  Gain : Gain  Gain=-1
  LMS Update : dspadpt3/LMS Update  Method=Normalized LMS  Length=200  NumFilters=1  StepSizeSource=Input port  StepSize=0.1  LeakageFactor=1.0  InitialConditions=0  AdaptiveFilterMode=Tapped delay-line FIR filter  EnableAdaptInput=off  EnableResetInput=off  SimulateUsing=Interpreted execution
  LMS filter copy : DiscreteFir  CoefSource=Input port
      settings: InputPortMap=u0,u1
  Primary path : DiscreteFir  Commented=through  Coefficients=conv([0.5 0.5 -.3 -.3 -.2 -.2],[.1 -.1 .2 -.2 .3 -.3 .15 -.15])
  Sec. path : DiscreteFir  Commented=through  Coefficients=[0.5 0.5 -.3 -.3 -.2 -.2]
  Sum : Sum  Inputs=++|
  y : Outport
  wires:
  Primary path/1 -> Sum/2  "Noise output (no ANC)"
  Gain/1 -> y/1, Sec. path/1
  Constant/1 -> LMS Update/3
  LMS filter copy/1 -> Gain/1
  [coefs] -> LMS filter copy/2
  Sum/1 -> LMS Update/2  "Error mic."
  Delay1/1 -> [coefs]
  LMS Update/1 -> Delay1/1
  In1/1 -> Primary path/1, Estim. sec. path/1, LMS filter copy/1
  Estim. sec. path/1 -> LMS Update/1
  Sec. path/1 -> Sum/1

== system samples10ANC/Audio Processing/Subsystem1/Subsystem8 ==
  note: Anti-noise
  In1 : Inport
  Constant : Constant  Value=0.5
  Delay1 : Delay  DelayLength=1
  Estim. sec. path : DiscreteFir  Commented=through  Coefficients="[0.466  0.533  -0.257  -0.274  -0.231  -0.175]"
  Gain : Gain  Gain=-1
  LMS Update : dspadpt3/LMS Update  Method=Normalized LMS  Length=200  NumFilters=1  StepSizeSource=Input port  StepSize=0.1  LeakageFactor=1.0  InitialConditions=0  AdaptiveFilterMode=Tapped delay-line FIR filter  EnableAdaptInput=off  EnableResetInput=off  SimulateUsing=Interpreted execution
  LMS filter copy : DiscreteFir  CoefSource=Input port
      settings: InputPortMap=u0,u1
  Primary path : DiscreteFir  Commented=through  Coefficients=conv([0.5 0.5 -.3 -.3 -.2 -.2],[.1 -.1 .2 -.2 .3 -.3 .15 -.15])
  Sec. path : DiscreteFir  Commented=through  Coefficients=[0.5 0.5 -.3 -.3 -.2 -.2]
  Sum : Sum  Inputs=++|
  y : Outport
  wires:
  Primary path/1 -> Sum/2  "Noise output (no ANC)"
  Gain/1 -> y/1, Sec. path/1
  Constant/1 -> LMS Update/3
  LMS filter copy/1 -> Gain/1
  [coefs] -> LMS filter copy/2
  Sum/1 -> LMS Update/2  "Error mic."
  Delay1/1 -> [coefs]
  LMS Update/1 -> Delay1/1
  In1/1 -> Primary path/1, Estim. sec. path/1, LMS filter copy/1
  Estim. sec. path/1 -> LMS Update/1
  Sec. path/1 -> Sum/1

== system samples10ANC/Audio Processing/Subsystem1/Subsystem9 ==
  note: Anti-noise
  In1 : Inport
  Constant : Constant  Value=0.5
  Delay1 : Delay  DelayLength=1
  Estim. sec. path : DiscreteFir  Commented=through  Coefficients="[0.466  0.533  -0.257  -0.274  -0.231  -0.175]"
  Gain : Gain  Gain=-1
  LMS Update : dspadpt3/LMS Update  Method=Normalized LMS  Length=200  NumFilters=1  StepSizeSource=Input port  StepSize=0.1  LeakageFactor=1.0  InitialConditions=0  AdaptiveFilterMode=Tapped delay-line FIR filter  EnableAdaptInput=off  EnableResetInput=off  SimulateUsing=Interpreted execution
  LMS filter copy : DiscreteFir  CoefSource=Input port
      settings: InputPortMap=u0,u1
  Primary path : DiscreteFir  Commented=through  Coefficients=conv([0.5 0.5 -.3 -.3 -.2 -.2],[.1 -.1 .2 -.2 .3 -.3 .15 -.15])
  Sec. path : DiscreteFir  Commented=through  Coefficients=[0.5 0.5 -.3 -.3 -.2 -.2]
  Sum : Sum  Inputs=++|
  y : Outport
  wires:
  Primary path/1 -> Sum/2  "Noise output (no ANC)"
  Gain/1 -> y/1, Sec. path/1
  Constant/1 -> LMS Update/3
  LMS filter copy/1 -> Gain/1
  [coefs] -> LMS filter copy/2
  Sum/1 -> LMS Update/2  "Error mic."
  Delay1/1 -> [coefs]
  LMS Update/1 -> Delay1/1
  In1/1 -> Primary path/1, Estim. sec. path/1, LMS filter copy/1
  Estim. sec. path/1 -> LMS Update/1
  Sec. path/1 -> Sum/1
